simulink model "SCARA_pd_control"  (R2022b)
settings: Solver=VariableStepAuto  StartTime=0.0  StopTime=T+1  FixedStep=0.01  RelTol=1e-3
settings Model: Creator=hyeonjae  LastModifiedBy=hyeonjae

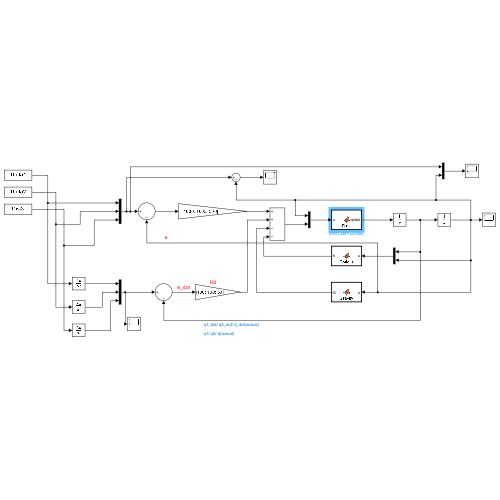
[thumbnail: Simulink's stored preview of the top-level diagram]
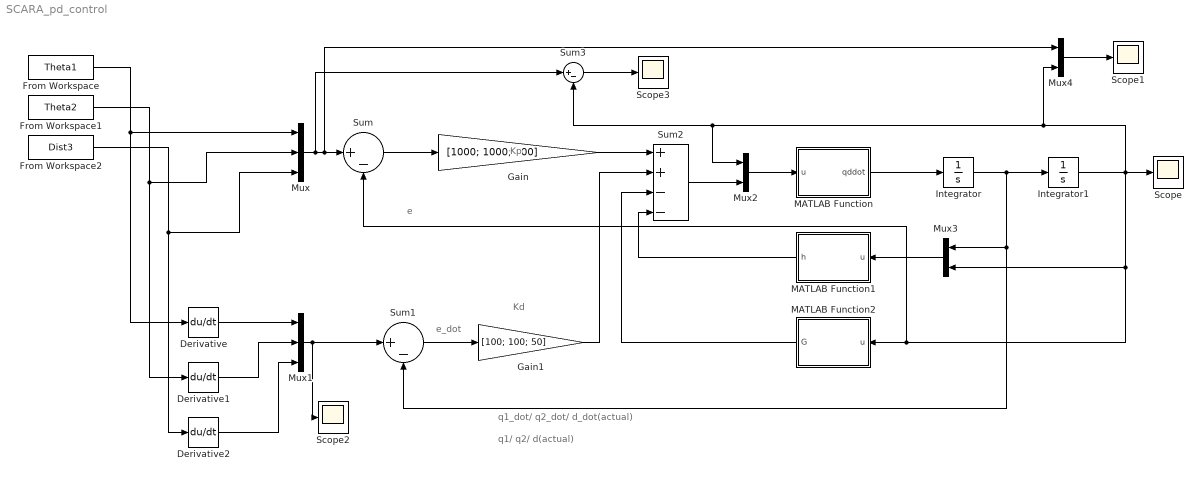
== system SCARA_pd_control ==
  note: Kp
  note: Kd
  note: q1/ q2/ d(actual)
  note: q1_dot/ q2_dot/ d_dot(actual)
  note: e
  note: e_dot
  Derivative : Derivative
  Derivative1 : Derivative
  Derivative2 : Derivative
  From Workspace : FromWorkspace  VariableName=Theta1  SampleTime=0.002
  From Workspace1 : FromWorkspace  VariableName=Theta2  SampleTime=0.002
  From Workspace2 : FromWorkspace  VariableName=Dist3  SampleTime=0.002
  Gain : Gain  Gain=[1000; 1000; 300]
  Gain1 : Gain  Gain=[100; 100; 50]
  Integrator : Integrator  InitialCondition=[0;0;0]
  Integrator1 : Integrator  InitialCondition=[0; 0; 0]
  MATLAB Function : MATLAB Function  TreatAsAtomicUnit=on
  MATLAB Function1 : MATLAB Function  TreatAsAtomicUnit=on
  MATLAB Function2 : MATLAB Function  TreatAsAtomicUnit=on
  Mux : Mux  Inputs=3
  Mux1 : Mux  Inputs=3
  Mux2 : Mux  Inputs=2
  Mux3 : Mux  Inputs=2
  Mux4 : Mux  Inputs=2
  Scope{,1..3} (4 alike) : Scope
  Sum : Sum  Inputs=|+-
  Sum1 : Sum  Inputs=|+-
  Sum2 : Sum  Inputs=++--
  Sum3 : Sum  Inputs=|+-
  wires:
  From Workspace/1 -> Derivative/1, Mux/1
  From Workspace1/1 -> Derivative1/1, Mux/2
  From Workspace2/1 -> Derivative2/1, Mux/3
  Derivative/1 -> Mux1/1
  Derivative1/1 -> Mux1/2
  Derivative2/1 -> Mux1/3
  Mux/1 -> Sum3/1, Mux4/1, Sum/1
  Mux1/1 -> Sum1/1, Scope2/1
  Sum/1 -> Gain/1
  Sum1/1 -> Gain1/1
  Gain1/1 -> Sum2/2
  Gain/1 -> Sum2/1
  Sum2/1 -> Mux2/2
  Mux2/1 -> MATLAB Function/1(u)
  MATLAB Function/1(qddot) -> Integrator/1
  Integrator/1 -> Mux3/1, Sum1/2, Integrator1/1
  Integrator1/1 -> Mux4/2, Sum3/2, Mux2/1, Sum/2, MATLAB Function2/1(u), Mux3/2, Scope/1
  Mux3/1 -> MATLAB Function1/1(u)
  MATLAB Function1/1(h) -> Sum2/4
  MATLAB Function2/1(G) -> Sum2/3
  Mux4/1 -> Scope1/1
  Sum3/1 -> Scope3/1

== matlab function SCARA_pd_control/MATLAB Function ==
  data: u input; qddot output
function qddot = Dinv(u)
m1=1; m2=1; m3=1; l1=1; l2=1;
q1=u(1); q2=u(2); d=u(3);

th1 = q1; th2 = q2;

% U
U11 = [-sin(th1) -cos(th1) 0 -l1*sin(th1); cos(th1) -sin(th1) 0 l1*cos(th1);
        0 0 0 0; 0 0 0 0];
U21 = [-sin(th1+th2) cos(th1+th2) 0 -l1*sin(th1)-l2*sin(th1+th2); 
        cos(th1+th2) sin(th1+th2) 0 l1*cos(th1)+l2*cos(th1+th2); 0 0 0 0; 0 0 0 0];
U22 = [-sin(th1+th2) cos(th1+th2) 0 -l2*sin(th1+th2); 
        cos(th1+th2) sin(th1+th2) 0 l2*cos(th1+th2); 0 0 0 0; 0 0 0 0];
U31 = [-sin(th1+th2) cos(th1+th2) 0 -l1*sin(th1)-l2*sin(th1+th2); 
        cos(th1+th2) sin(th1+th2) 0 l1*cos(th1)+l2*cos(th1+th2); 0 0 0 0; 0 0 0 0];
U32 = [-sin(th1+th2) cos(th1+th2) 0 -l2*sin(th1+th2); 
        cos(th1+th2) sin(th1+th2) 0 l2*cos(th1+th2); 0 0 0 0; 0 0 0 0];
U33 = [0 0 0 0; 0 0 0 0; 0 0 0 -1; 0 0 0 0];
    
% J
J1 = [m1*l1^2/3 0 0 -m1*l1/2; 0 0 0 0; 0 0 0 0; -m1*l1/2 0 0 m1];
J2 = [m2*l2^2/3 0 0 -m2*l2/2; 0 0 0 0; 0 0 0 0; -m2*l2/2 0 0 m2];
J3 = [0 0 0 0; 0 0 0 0; 0 0 m3*d^2/3 -m3*d/2; 0 0 -m3*d/2 m3];

% d
d11 = trace(U11*J1*transpose(U11)) + trace(U21*J2*transpose(U21)) + trace(U31*J3*transpose(U31));  
d12 = trace(U22*J2*transpose(U21)) + trace(U32*J3*transpose(U31)); 
d13 = trace(U33*J3*transpose(U31));
d21 = trace(U21*J2*transpose(U22)) + trace(U31*J3*transpose(U32));
d22 = trace(U22*J2*transpose(U22)) + trace(U32*J3*transpose(U32));
d23 = trace(U33*J3*transpose(U32));
d31 = trace(U31*J3*transpose(U33));
d32 = trace(U32*J3*transpose(U33));
d33 = trace(U33*J3*transpose(U33));

D=[d11 d12 d13; d21 d22 d23; d31 d32 d33];
D_inv= inv(D);
C_input= [u(4); u(5); u(6)];
qddot = (D_inv*C_input);

== matlab function SCARA_pd_control/MATLAB Function2 ==
  data: u input; G output
function G = Gravity(u)

m1=1; m2=1; m3=1; l1=1; l2=1; g=9.8;
q1= u(1); q2=u(2); d=u(3);


th1 = q1; th2 = q2;
% U
U11 = [-sin(th1) -cos(th1) 0 -l1*sin(th1); cos(th1) -sin(th1) 0 l1*cos(th1);
        0 0 0 0; 0 0 0 0];
U21 = [-sin(th1+th2) cos(th1+th2) 0 -l1*sin(th1)-l2*sin(th1+th2); 
        cos(th1+th2) sin(th1+th2) 0 l1*cos(th1)+l2*cos(th1+th2); 0 0 0 0; 0 0 0 0];
U22 = [-sin(th1+th2) cos(th1+th2) 0 -l2*sin(th1+th2); 
        cos(th1+th2) sin(th1+th2) 0 l2*cos(th1+th2); 0 0 0 0; 0 0 0 0];
U31 = [-sin(th1+th2) cos(th1+th2) 0 -l1*sin(th1)-l2*sin(th1+th2); 
        cos(th1+th2) sin(th1+th2) 0 l1*cos(th1)+l2*cos(th1+th2); 0 0 0 0; 0 0 0 0];
U32 = [-sin(th1+th2) cos(th1+th2) 0 -l2*sin(th1+th2); 
        cos(th1+th2) sin(th1+th2) 0 l2*cos(th1+th2); 0 0 0 0; 0 0 0 0];
U33 = [0 0 0 0; 0 0 0 0; 0 0 0 -1; 0 0 0 0];

R11 = [-l1/2; 0; 0; 1]; 
R22 = [-l2/2; 0; 0; 1];   
R33 = [0; 0; -d/2; 1];
g1 = [0 0 -g 0];
g2 = g1;
g3 = [0 0 g 0];
    
G1 = -m1*g1*U11*R11 -m2*g2*U21*R22 -m3*g3*U31*R33;   
G2 = -m2*g2*U22*R22 -m3*g3*U32*R33;   
G3 = -m3*g3*U33*R33;
 
G = [G1; G2; G3];

== matlab function SCARA_pd_control/MATLAB Function1 ==
  data: u input; h output
function h = Coriolis(u)

dotq1=u(1); dotq2=u(2); dotd=u(3); q1=u(4); q2=u(5); d=u(6);
m1=1; m2=1; m3=1; l1=1; l2=1;

th1 = q1; th2 = q2;
th_p1 = dotq1; th_p2 = dotq2;
A01 = [cos(th1) -sin(th1) 0 l1*cos(th1); sin(th1) cos(th1) 0 l1*sin(th1);
            0 0 1 0; 0 0 0 1];
A12 = [cos(th2) sin(th2) 0 l2*cos(th2); sin(th2) -cos(th2) 0 l2*sin(th2);
        0 0 -1 0; 0 0 0 1];
A23 = [1 0 0 0; 0 1 0 0; 0 0 1 d; 0 0 0 1];
A02 = A01*A12;
A13 = A12*A23;
A03 = A01*A12*A23;

Q1 = [0 -1 0 0; 1 0 0 0; 0 0 0 0; 0 0 0 0]; Q2 = Q1;
Q3 = [0 0 0 0; 0 0 0 0; 0 0 0 1; 0 0 0 0];


% U
U11 = [-sin(th1) -cos(th1) 0 -l1*sin(th1); cos(th1) -sin(th1) 0 l1*cos(th1);
        0 0 0 0; 0 0 0 0];
U21 = [-sin(th1+th2) cos(th1+th2) 0 -l1*sin(th1)-l2*sin(th1+th2); 
        cos(th1+th2) sin(th1+th2) 0 l1*cos(th1)+l2*cos(th1+th2); 0 0 0 0; 0 0 0 0];
U22 = [-sin(th1+th2) cos(th1+th2) 0 -l2*sin(th1+th2); 
        cos(th1+th2) sin(th1+th2) 0 l2*cos(th1+th2); 0 0 0 0; 0 0 0 0];
U31 = [-sin(th1+th2) cos(th1+th2) 0 -l1*sin(th1)-l2*sin(th1+th2); 
        cos(th1+th2) sin(th1+th2) 0 l1*cos(th1)+l2*cos(th1+th2); 0 0 0 0; 0 0 0 0];
U32 = [-sin(th1+th2) cos(th1+th2) 0 -l2*sin(th1+th2); 
        cos(th1+th2) sin(th1+th2) 0 l2*cos(th1+th2); 0 0 0 0; 0 0 0 0];
U33 = [0 0 0 0; 0 0 0 0; 0 0 0 -1; 0 0 0 0];

% U - 3
U111 = Q1*Q1*A01;
U211 = Q1*Q1*A02;
U212 = Q1*A01*Q2*A12;
U221 = Q1*A01*Q2*A12;
U222 = A01*Q2*Q2*A12;
U311 = Q1*Q1*A03;
U312 = Q1*A01*Q2*A13;
U321 = Q1*A01*Q2*A13;
U322 = A01*Q2*Q2*A13;

% J
J1 = [m1*l1^2/3 0 0 -m1*l1/2; 0 0 0 0; 0 0 0 0; -m1*l1/2 0 0 m1];
J2 = [m2*l2^2/3 0 0 -m2*l2/2; 0 0 0 0; 0 0 0 0; -m2*l2/2 0 0 m2];
J3 = [0 0 0 0; 0 0 0 0; 0 0 m3*d^2/3 -m3*d/2; 0 0 -m3*d/2 m3];

% h1
H111 = trace(U111*J1*transpose(U11)) + trace(U211*J2*transpose(U21)) + trace(U311*J3*transpose(U31));
H112 = trace(U212*J2*transpose(U21)) + trace(U312*J3*transpose(U31));
H121 = trace(U221*J2*transpose(U21)) + trace(U321*J3*transpose(U31));
H122 = trace(U222*J2*transpose(U21)) + trace(U322*J3*transpose(U31));
h1 = H111*th_p1*th_p1 + H112*th_p1*th_p2 + H121*th_p2*th_p1 + H122*th_p2*th_p2;

% h2 
H211 = trace(U211*J2*transpose(U22)) + trace(U311*J3*transpose(U32));
H212 = trace(U212*J2*transpose(U22)) + trace(U312*J3*transpose(U32));
H221 = trace(U221*J2*transpose(U22)) + trace(U321*J3*transpose(U32));
H222 = trace(U222*J2*transpose(U22)) + trace(U322*J3*transpose(U32));
h2 = H211*th_p1*th_p1 + H212*th_p1*th_p2 + H221*th_p2*th_p1 + H222*th_p2*th_p2;

% h3
h3 = 0;

h = [h1; h2; h3];
